simulink model "cube"  (R2014b)
settings: Solver=ode45  StartTime=0.0  StopTime=10.0  RelTol=1e-3
values from neighbouring files (symbols this model uses):
  A = [a11, a12, a13; a21, a22, a23; a31, a32, a33]    [gs.m]
  B = [b1; b2; b3]    [gs.m]
  C = [1 0 0; 0 1 0; 0 0 1]    [gs.m]
  D = [0; 0; 0]    [gs.m]
  X0 = x0    [gs.m]
undefined symbols (not defined in the file or in its folder): K
settings Model: Creator=MikaelSjostedt  LastModifiedBy=MikaelSjostedt

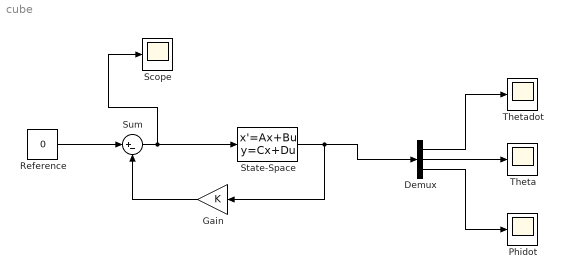
== system cube ==
  Demux : Demux  Outputs=3
  Gain : Gain  Gain=K
  "Phidot " : Scope
      settings: SaveName=ScopeData3
  "Reference " : Constant  Value=0
  Scope : Scope
  State-Space : StateSpace  A=A  B=B  C=C  D=D  X0=X0
  Sum : Sum  Inputs=|+-
  "Theta " : Scope
  Thetadot : Scope
      settings: SaveName=ScopeData2
  wires:
  "Reference "/1 -> Sum/1
  Sum/1 -> Scope/1, State-Space/1
  Demux/2 -> "Theta "/1
  Demux/1 -> Thetadot/1
  Demux/3 -> "Phidot "/1
  State-Space/1 -> Gain/1, Demux/1
  Gain/1 -> Sum/2
